simulink model "FM"  (R2020b)
settings: Solver=VariableStepAuto  StartTime=0.0  StopTime=10.0  MaxStep=0.001  RelTol=1e-3
settings Model: Creator=MEDIA  LastModifiedBy=MEDIA

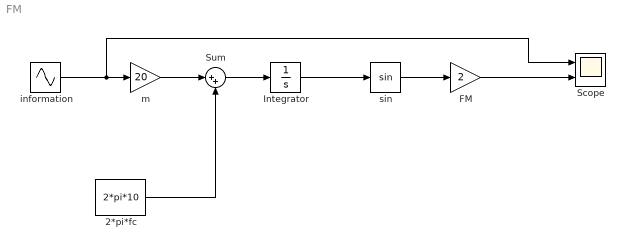
== system FM ==
  2*pi*fc : Constant  Value=2*pi*10
  FM : Gain  Gain=2
  Integrator : Integrator
  Scope : Scope  NumInputPorts=2
  Sum : Sum  Inputs=|++
  information : Sin  Frequency=2*pi  SampleTime=0
  m : Gain  Gain=20
  sin : Trigonometry
  wires:
  information/1 -> Scope/1, m/1
  m/1 -> Sum/1
  Sum/1 -> Integrator/1
  2*pi*fc/1 -> Sum/2
  Integrator/1 -> sin/1
  sin/1 -> FM/1
  FM/1 -> Scope/2
